simulink model "template_general"  (R2017a)
settings: Solver=VariableStepAuto  StartTime=0.0  StopTime=10.0  RelTol=1e-3
values from neighbouring files (symbols this model uses):
  filter_pole = 30    [Init_SNR_sim.m]
  step_period = 1    [Init_SNR_sim.m]
undefined symbols (not defined in the file or in its folder): magnitude
settings Model: Creator=ignacio  LastModifiedBy=ignacio

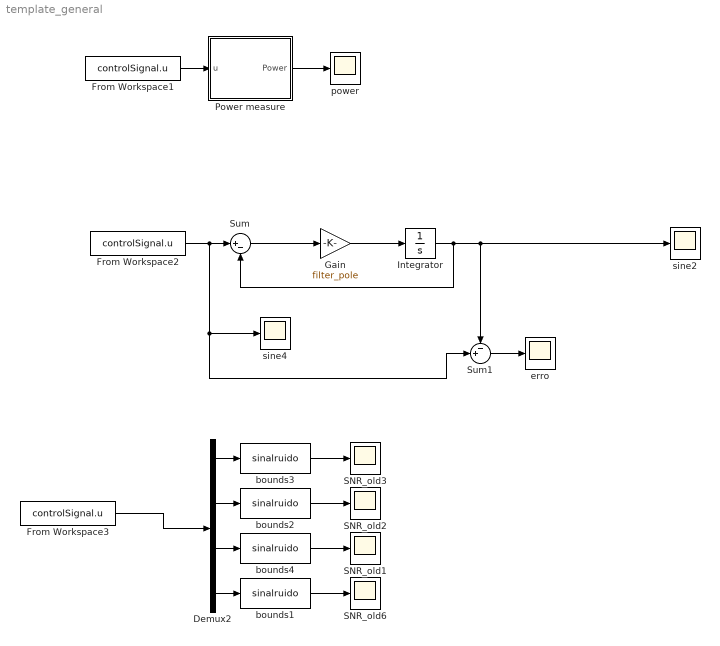
== system template_general ==
  Demux2 : Demux
  From Workspace1 : FromWorkspace  VariableName=controlSignal.u  SampleTime=0
  From Workspace2 : FromWorkspace  VariableName=controlSignal.u  SampleTime=0
  From Workspace3 : FromWorkspace  VariableName=controlSignal.u  SampleTime=0
  Gain : Gain  Gain=filter_pole
  Integrator : Integrator
  Power measure : Subsystem  mask(Measure power){window=0.1, sampling=1e-3}
      mask prompts: window "Window Length"
      mask help: Foo bar
      mask init:
      | global step_period;
      | 
      | N = step_period / window;
  SNR_old{1..3,6} (4 alike) : Scope
  Sum : Sum  Inputs=|+-
  Sum1 : Sum  Inputs=-+|
  bounds{1..4} (4 alike) : MATLABFcn  MATLABFcn=sinalruido  Output1D=off
  erro : Scope
  power : Scope
  sine2 : Scope
  sine4 : Scope
  wires:
  From Workspace2/1 -> Sum1/2, sine4/1, Sum/1
  Integrator/1 -> sine2/1, Sum1/1, Sum/2
  Sum/1 -> Gain/1
  Power measure/1(Power) -> power/1
  Gain/1 -> Integrator/1
  Sum1/1 -> erro/1
  bounds1/1 -> SNR_old6/1
  From Workspace3/1 -> Demux2/1
  From Workspace1/1 -> Power measure/1(u)
  Demux2/2 -> bounds2/1
  Demux2/1 -> bounds3/1
  Demux2/3 -> bounds4/1
  Demux2/4 -> bounds1/1
  bounds4/1 -> SNR_old1/1
  bounds2/1 -> SNR_old2/1
  bounds3/1 -> SNR_old3/1

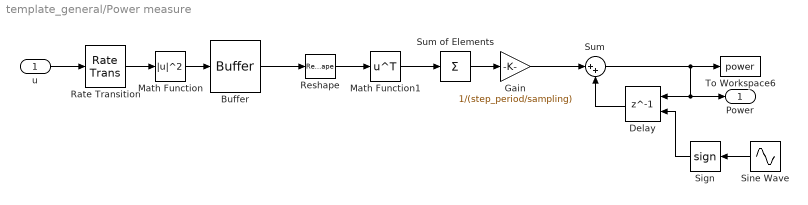
== system template_general/Power measure ==
  u : Inport
  Buffer : Buffer  N=5 * window/sampling  OutputFrames=off
  Delay : Delay  DelayLength=1  ExternalReset=Either
      settings: InputPortMap=u0,r5
  Gain : Gain  Gain=1/(step_period/sampling)
  Math Function : Math  Operator=magnitude^2  SaturateOnIntegerOverflow=on
  Math Function1 : Math  Operator=transpose  SaturateOnIntegerOverflow=on
  Rate Transition : RateTransition  OutPortSampleTime=sampling
  Reshape : Reshape  OutputDimensionality=Customize  OutputDimensions=[5,window/sampling]
  Sign : Signum
  Sine Wave : Sin  Frequency=2*pi / (2 * step_period)  SampleTime=window
  Sum : Sum  Inputs=|++
  Sum of Elements : Sum  Inputs=+  CollapseMode=Specified dimension
  To Workspace6 : ToWorkspace  VariableName=power  SaveFormat=Timeseries  SampleTime=-1
  Power : Outport
  wires:
  Math Function/1 -> Buffer/1
  Rate Transition/1 -> Math Function/1
  Gain/1 -> Sum/1
  Reshape/1 -> Math Function1/1
  Sum of Elements/1 -> Gain/1
  Buffer/1 -> Reshape/1
  Math Function1/1 -> Sum of Elements/1
  Sum/1 -> Delay/1, Power/1, To Workspace6/1
  Delay/1 -> Sum/2
  Sine Wave/1 -> Sign/1
  Sign/1 -> Delay/2
  u/1 -> Rate Transition/1
